simulink model "mass_spring3"  (R2022b)
settings: Solver=VariableStepAuto  StartTime=0.0  StopTime=Sim_Tim  RelTol=1e-3
undefined symbols (not defined in the file): b, F, k, m
settings Model: Creator=HashimAbdulAzizHashi  LastModifiedBy=HashimAbdulAzizHashi

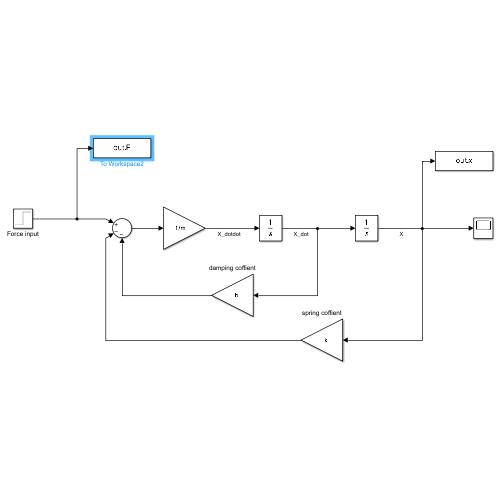
[thumbnail: Simulink's stored preview of the top-level diagram]
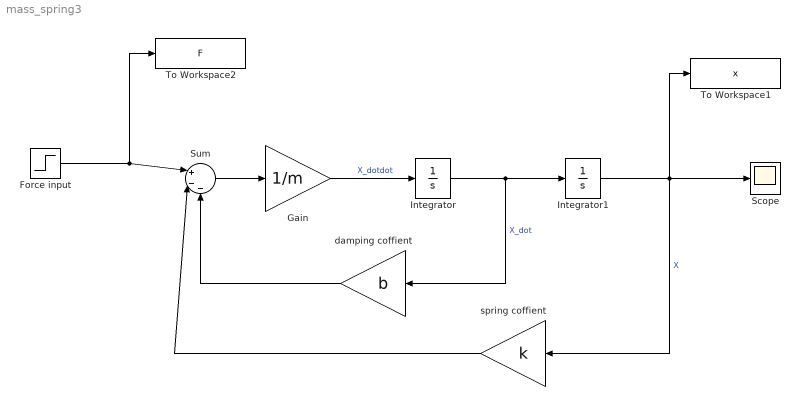
== system mass_spring3 ==
  Force input : Step  After=F  SampleTime=0
  Gain : Gain  Gain=1/m
  Integrator : Integrator
  Integrator1 : Integrator
  Scope : Scope
  Sum : Sum  Inputs=|+--
  To Workspace1 : ToWorkspace  VariableName=x  SaveFormat=Timeseries  SampleTime=-1
  To Workspace2 : ToWorkspace  VariableName=F  SaveFormat=Timeseries  SampleTime=-1
  damping coffient : Gain  Gain=b
  spring coffient : Gain  Gain=k
  wires:
  Integrator/1 -> damping coffient/1, Integrator1/1  "X_dot"
  Gain/1 -> Integrator/1  "X_dotdot"
  Integrator1/1 -> spring coffient/1, To Workspace1/1, Scope/1  "X"
  damping coffient/1 -> Sum/3
  spring coffient/1 -> Sum/2
  Force input/1 -> To Workspace2/1, Sum/1
  Sum/1 -> Gain/1
